simulink subsystem "R2216_810KV_Model"  (R2024a)
settings: Solver=VariableStepAuto  StartTime=0.0  StopTime=10.0  RelTol=1e-3
settings Model: Creator=UASG  LastModifiedBy=UASG

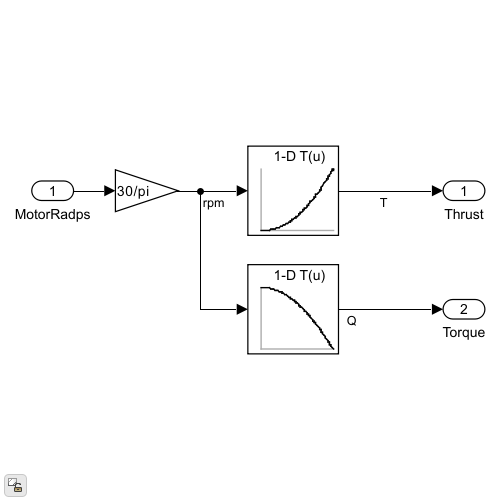
[thumbnail: Simulink's stored preview of the top-level diagram]
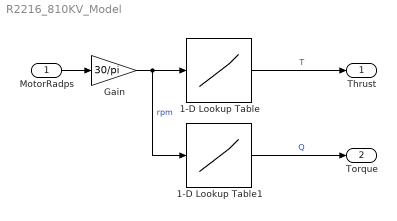
== system R2216_810KV_Model ==
  MotorRadps : Inport
  1-D Lookup Table : Lookup_n-D  NumberOfTableDimensions=1  BreakpointsForDimension1=[0;1096.20419851365;1227.36627002605;1352.02920708404;1495.06014385177;1620.44566028244;1748.45134656175;1878.92697495564;2004.98392630248;2132.98465841792;2258.64935655418;2371.31855428499;2497.8308515765;2618.61861250699;2737.72458051162;2858.55080906752;2971.03597418133;3079.46134770783;3197.69101154887;3305.56006161401;3411.72691925497;3530.31182578819;3632.73012990194;3734.18616053774;3843.41469145528;3943.22098551972;4038.70870578957;4138.74755413486;4239.58140007187;4352.366437811;4453.33754322957;4565.87341566777;4661.7338639141;4770.88167110257;4877.4533130745;4970.90137493364;5086.30017125052;5183.23392452993;5278.93146821109;5375.73991028653;5467.57029192882;5566.59470236474;5667.0698085527;5744.84668438018;5849.28045892805;5947.41311986594;6038.5242734817;6135.1776793699;6222.0597255623;6319.10771603231;6402.00661446681;6486.15221367013;6572.77081491278;6657.06212481839;6733.08231241901;6819.53072356138;6897.45505861957;6980.27119337517;7057.8807933164;7133.66959232178;7214.1683440681;7292.41324267134;7357.83559947274;7433.94904192282;7515.14137661206;7586.69349123755;7652.23125091516;7722.12867480541;7792.32101715709;7868.54461689811;7931.14718018873;7990.32495913264;8049.03996088606;8117.93256377328;8196.33016719253;8261.68200001402;8332.67866544236;8390.0035870959;8443.94860329904;8494.21238431943;8562.43355229049;8620.20026879339;8681.81025077998;8729.31193972769;8792.00600933935;8833.29634246969;8849.66023718007]  Table=[0;0.076257457969369;0.0953020471386153;0.121381171421294;0.136609957132142;0.199555167932659;0.209438659984919;0.239293679694445;0.272072826396254;0.31294293932726;0.349400772638769;0.393213239215274;0.446558364551759;0.488921395248075;0.539466882825021;0.601390686274775;0.652637125665564;0.705227214870823;0.757109681068905;0.824514465484516;0.872723129339445;0.959180603659065;1.00022083202008;1.05651807953516;1.15229187534522;1.22088103483446;1.2783140530146;1.33205146834479;1.41450575015041;1.49278124410321;1.56118480146363;1.66802658352804;1.76744999860542;1.84332696029787;1.90524897682083;1.97502513220966;2.07595075707163;2.15706913241219;2.2479286413044;2.32362071563874;2.43190657280298;2.52920354500526;2.62429139918649;2.731473173854;2.80173465855785;2.92322804898129;3.04359448424515;3.09804571726205;3.1422623866775;3.2577440788797;3.33201876288755;3.47938256454509;3.48601754282921;3.59880264338319;3.79853531270991;3.85416829997448;3.90116018581673;4.06471592672266;4.03970514640099;4.21337489291455;4.23658302149471;4.33753533113002;4.51971370822685;4.65243424051702;4.71023298304598;4.7922729360942;4.97128440241278;5.01603095518445;5.14052018792851;5.17025417313041;5.17833680036794;5.3016180706048;5.44462701255689;5.5450599221398;5.60297922266258;5.70261683069735;5.75583579900276;5.89585652285519;5.98116821971975;6.14282886520512;6.14129639679361;6.19064893204836;6.4143716891167;6.4443353539748;6.42359651995572;6.57378033033815;6.43574571604392]  InternalRulePriority=Speed  RndMeth=Simplest
  1-D Lookup Table1 : Lookup_n-D  NumberOfTableDimensions=1  BreakpointsForDimension1=[0;1096.20419851365;1227.36627002605;1352.02920708404;1495.06014385177;1620.44566028244;1748.45134656175;1878.92697495564;2004.98392630248;2132.98465841792;2258.64935655418;2371.31855428499;2497.8308515765;2618.61861250699;2737.72458051162;2858.55080906752;2971.03597418133;3079.46134770783;3197.69101154887;3305.56006161401;3411.72691925497;3530.31182578819;3632.73012990194;3734.18616053774;3843.41469145528;3943.22098551972;4038.70870578957;4138.74755413486;4239.58140007187;4352.366437811;4453.33754322957;4565.87341566777;4661.7338639141;4770.88167110257;4877.4533130745;4970.90137493364;5086.30017125052;5183.23392452993;5278.93146821109;5375.73991028653;5467.57029192882;5566.59470236474;5667.0698085527;5744.84668438018;5849.28045892805;5947.41311986594;6038.5242734817;6135.1776793699;6222.0597255623;6319.10771603231;6402.00661446681;6486.15221367013;6572.77081491278;6657.06212481839;6733.08231241901;6819.53072356138;6897.45505861957;6980.27119337517;7057.8807933164;7133.66959232178;7214.1683440681;7292.41324267134;7357.83559947274;7433.94904192282;7515.14137661206;7586.69349123755;7652.23125091516;7722.12867480541;7792.32101715709;7868.54461689811;7931.14718018873;7990.32495913264;8049.03996088606;8117.93256377328;8196.33016719253;8261.68200001402;8332.67866544236;8390.0035870959;8443.94860329904;8494.21238431943;8562.43355229049;8620.20026879339;8681.81025077998;8729.31193972769;8792.00600933935;8833.29634246969;8849.66023718007]  Table=[0;-0.00225694477558136;-0.00278683006763458;-0.00348073244094849;-0.0041835606098175;-0.00500018894672394;-0.00575312972068787;-0.00639994442462921;-0.00704078376293182;-0.00780700147151947;-0.00884990394115448;-0.00978416204452515;-0.0107143968343735;-0.0120534598827362;-0.013313889503479;-0.0146090239286423;-0.0157379060983658;-0.0169038623571396;-0.0181442201137543;-0.0193782448768616;-0.0204462110996246;-0.022020161151886;-0.0233710408210754;-0.0245336890220642;-0.0259430557489395;-0.0274340808391571;-0.0288791954517365;-0.0301083475351334;-0.0317321568727493;-0.0330489128828049;-0.0346760898828506;-0.0356295853853226;-0.0386059731245041;-0.0397168397903442;-0.0413920730352402;-0.0434082001447678;-0.0446431040763855;-0.0463967323303223;-0.0485915243625641;-0.0501280128955841;-0.0519890785217285;-0.0535075068473816;-0.0558752119541168;-0.0575185716152191;-0.0593845844268799;-0.0611693561077118;-0.063087671995163;-0.0643691420555115;-0.0663736164569855;-0.0682030022144318;-0.0703082382678986;-0.0723428130149841;-0.0740454792976379;-0.0758231580257416;-0.0782356262207031;-0.0793281197547913;-0.0809338390827179;-0.0827755033969879;-0.0845003128051758;-0.0865840017795563;-0.0880957543849945;-0.0897682905197144;-0.092194527387619;-0.0942575931549072;-0.0956821441650391;-0.0977562963962555;-0.100761204957962;-0.101732224225998;-0.103003293275833;-0.104814499616623;-0.106198281049728;-0.10841953754425;-0.109262079000473;-0.111167639493942;-0.113433569669724;-0.114739984273911;-0.116187691688538;-0.11840695142746;-0.120427638292313;-0.121266633272171;-0.123398423194885;-0.125064343214035;-0.126681536436081;-0.12694725394249;-0.128406554460526;-0.13033264875412;-0.128643214702606]  InternalRulePriority=Speed  RndMeth=Simplest
  Gain : Gain  Gain=30/pi
  Thrust : Outport
  Torque : Outport  Port=2
  wires:
  MotorRadps/1 -> Gain/1
  Gain/1 -> 1-D Lookup Table1/1, 1-D Lookup Table/1  "rpm"
  1-D Lookup Table/1 -> Thrust/1  "T"
  1-D Lookup Table1/1 -> Torque/1  "Q"
